simulink model "sampled_data_eul_gain"  (R2020b)
settings: Solver=ode45  StartTime=0.0  StopTime=10.0  MaxStep=0.5e-3  RelTol=1e-6
values from neighbouring files (symbols this model uses):
  s_star = C_features_desired(:)    [init.m]
  Ts = 0.1    [init.m]
settings Model: Creator=marco  LastModifiedBy=marco

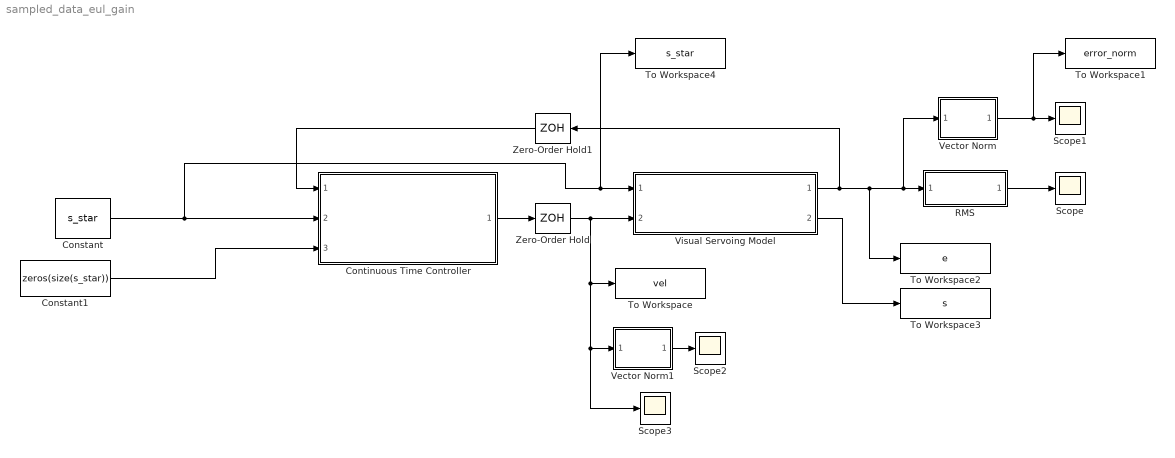
== system sampled_data_eul_gain ==
  Constant : Constant  Value=s_star
  Constant1 : Constant  Value=zeros(size(s_star))
  Continuous Time Controller : Subsystem  ReferencedSubsystem=continuous_time_controller  lambda=lambda  forward_action_enabled=off
  RMS : Subsystem  ReferencedSubsystem=RMS
  Scope{,1..3} (4 alike) : Scope
  To Workspace : ToWorkspace  VariableName=vel  SaveFormat=Timeseries  SampleTime=-1
  To Workspace1 : ToWorkspace  VariableName=error_norm  SaveFormat=Timeseries  SampleTime=-1
  To Workspace2 : ToWorkspace  VariableName=e  SaveFormat=Timeseries  SampleTime=Ts
  To Workspace3 : ToWorkspace  VariableName=s  SaveFormat=Timeseries  SampleTime=Ts
  To Workspace4 : ToWorkspace  VariableName=s_star  SaveFormat=Timeseries  SampleTime=Ts
  Vector Norm : Subsystem  ReferencedSubsystem=Norm
  Vector Norm1 : Subsystem  ReferencedSubsystem=Norm
  Visual Servoing Model : Subsystem  ReferencedSubsystem=Features_System  s0=s0  noise_perc=0  noise_sample_time=1
  Zero-Order Hold : ZeroOrderHold  SampleTime=Ts
  Zero-Order Hold1 : ZeroOrderHold  SampleTime=Ts
  wires:
  Continuous Time Controller/1 -> Zero-Order Hold/1
  Constant/1 -> To Workspace4/1, Visual Servoing Model/1, Continuous Time Controller/2
  Constant1/1 -> Continuous Time Controller/3
  Zero-Order Hold1/1 -> Continuous Time Controller/1
  Visual Servoing Model/1 -> Zero-Order Hold1/1, To Workspace2/1, Vector Norm/1, RMS/1
  RMS/1 -> Scope/1
  Vector Norm/1 -> To Workspace1/1, Scope1/1
  Vector Norm1/1 -> Scope2/1
  Zero-Order Hold/1 -> To Workspace/1, Scope3/1, Vector Norm1/1, Visual Servoing Model/2
  Visual Servoing Model/2 -> To Workspace3/1
